simulink model "Pendulo_001"  (R2020a)
settings: Solver=VariableStepAuto  StartTime=0.0  StopTime=10.0  RelTol=1e-3
settings Model: Creator=Win10  LastModifiedBy=Win10

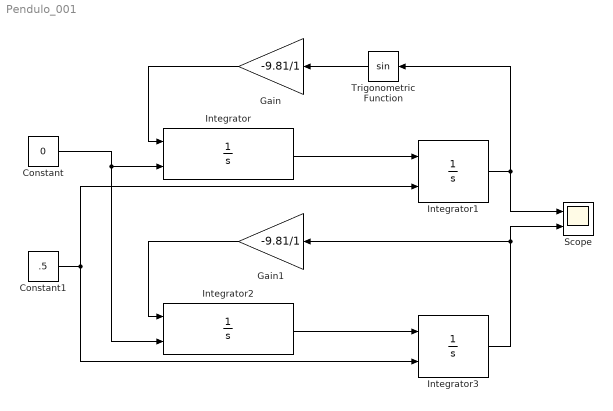
== system Pendulo_001 ==
  Constant : Constant  Value=0
  Constant1 : Constant  Value=.5
  Gain : Gain  Gain=-9.81/1
  Gain1 : Gain  Gain=-9.81/1
  Integrator{,1..3} (4 alike) : Integrator  InitialConditionSource=external
  Scope : Scope  NumInputPorts=2
  Trigonometric Function : Trigonometry
  wires:
  Integrator/1 -> Integrator1/1
  Integrator1/1 -> Scope/1, Trigonometric Function/1
  Gain/1 -> Integrator/1
  Trigonometric Function/1 -> Gain/1
  Constant1/1 -> Integrator1/2, Integrator3/2
  Constant/1 -> Integrator2/2, Integrator/2
  Integrator3/1 -> Gain1/1, Scope/2
  Gain1/1 -> Integrator2/1
  Integrator2/1 -> Integrator3/1
